simulink model "DAB_cc_2023a"  (R2023a)
settings: Solver=VariableStepAuto  StartTime=0.0  StopTime=0.3  RelTol=1e-3
undefined symbols (not defined in the file): Ion, Lithium
libraries: spsMosfetLib x8, spsVoltageMeasurementLib x6, spsSeriesRLCBranchLib x4, spsMeanLib x3, spsCurrentMeasurementLib x3, slpidlib x2, spsBatteryLib x1, spsDCVoltageSourceLib x1, spsLinearTransformerLib x1, spsRMSLib x1, eeGeneralControl x1, spspowerguiLib x1
settings Model: Creator=saivi  LastModifiedBy=saivi
settings RTWCC: GPUComputeCapability=5.0
settings ConfigComp: CovBoundaryAbsTol=1.0e-5

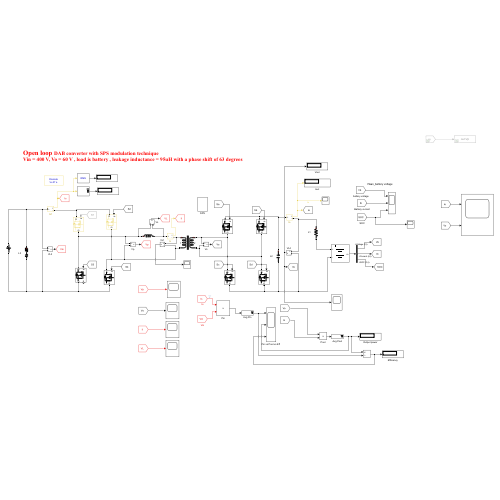
[thumbnail: Simulink's stored preview of the top-level diagram]
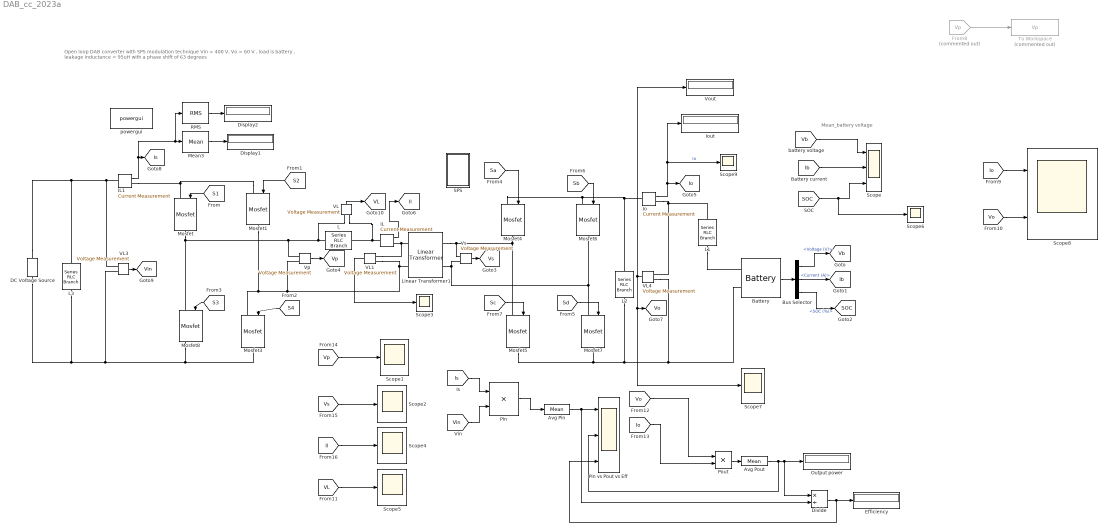
== system DAB_cc_2023a ==
  note: Open loop DAB converter with SPS modulation technique
      | Vin = 400 V, Vo = 60 V , load is battery , leakage inductance = 95uH with a phase shift of 63 degrees
  note: Mean_battery voltage
  Avg Pin : spsMeanLib/Mean  Freq=50000  Vinit=0  Ts=1e-7
  Avg Pout : spsMeanLib/Mean  Freq=50000  Vinit=0  Ts=1e-7
  Battery : spsBatteryLib/Battery  BatType=Lithium-Ion  NomV=48  NomQ=120  SOC=60  Batt_Tr=0.1  PresetModel=on  MaxQ=120  MinV=36  FullV=55.8714  Dis_rate=52.1739  R=0.004  Normal_OP=108.5217  expZone="[51.8585      5.89565]"
  Bus Selector : BusSelector  OutputSignals=Voltage (V),Current (A),SOC (%)
  DC Voltage Source : spsDCVoltageSourceLib/DC Voltage Source  Amplitude=400  Measurements=None
  Display1 : Display
  Display2 : Display
  Divide : Product  Inputs=*/
  Efficiency : Display
  From8 : From  Commented=on  GotoTag=Vp  TagVisibility=global
  IL : spsCurrentMeasurementLib/Current Measurement  PhasorSimulation=off  OutputType=Complex  PSBequivalent=0
  IL1 : spsCurrentMeasurementLib/Current Measurement  PhasorSimulation=off  OutputType=Complex  PSBequivalent=0
  Io : spsCurrentMeasurementLib/Current Measurement  PhasorSimulation=off  OutputType=Complex  PSBequivalent=0
  Iout : Display
  L : spsSeriesRLCBranchLib/Series RLC Branch  LConnTagsString=__new0  RConnTagsString=__new0  BranchType=L  Resistance=1  Inductance=90e-6  SetiL0=off  InitialCurrent=0  Capacitance=1e-6  Setx0=off  InitialVoltage=0  Measurements=None
  L1 : spsSeriesRLCBranchLib/Series RLC Branch  LConnTagsString=__new0  RConnTagsString=__new0  BranchType=R  Resistance=0.01  Inductance=19.108e-6*2  SetiL0=off  InitialCurrent=0  Capacitance=1000e-6  Setx0=off  InitialVoltage=0  Measurements=None
  L2 : spsSeriesRLCBranchLib/Series RLC Branch  LConnTagsString=__new0  RConnTagsString=__new0  BranchType=C  Resistance=0.8  Inductance=19.108e-6*2  SetiL0=off  InitialCurrent=0  Capacitance=1200e-6  Setx0=off  InitialVoltage=0  Measurements=None
  L3 : spsSeriesRLCBranchLib/Series RLC Branch  LConnTagsString=__new0  RConnTagsString=__new0  BranchType=RC  Resistance=0.8  Inductance=19.108e-6*2  SetiL0=off  InitialCurrent=0  Capacitance=1200e-6  Setx0=off  InitialVoltage=0  Measurements=None
  Linear Transformer1 : spsLinearTransformerLib/Linear Transformer  UNITS=SI  NominalPower=[1500 50000 ]  winding1=[400 0 0]  winding2=[60 0 0]  ThreeWindings=off  winding3=[3.15e+05 0.7938 0.084225]  RmLm=[5000 5866]  Measurements=None  DataType=on
  Mean3 : spsMeanLib/Mean  Freq=15000  Vinit=0  Ts=1e-6
  Mosfet{,1,3..7} (7 alike) : spsMosfetLib/Mosfet  Ron=0.01  Lon=0  Rd=0.01  Vfd=0  IC=0  Rs=1e5  Cs=inf  Measurements=off
  Mosfet8 : spsMosfetLib/Mosfet  Ron=0.01  Lon=0  Rd=0.01  Vfd=0  IC=0  Rs=1e5  Cs=inf  Measurements=on
  Output power : Display
  Pin : Product
  "Pin vs Pout vs Eff " : Scope  NumInputPorts=3
  Pout : Product
  RMS : spsRMSLib/RMS  TrueRMS=on  Freq=60  RMSInit=120  Ts=0
  SPS : Subsystem
  Scope : Scope  NumInputPorts=3
  Scope{1..7,9} (8 alike) : Scope
  Scope8 : Scope  NumInputPorts=2
  To Workspace : ToWorkspace  Commented=on  VariableName=Vp  SaveFormat=Structure With Time  SampleTime=-1
  VL{,1,3..4} (4 alike) : spsVoltageMeasurementLib/Voltage Measurement  PhasorSimulation=off  OutputType=Complex  PSBequivalent=0
  Vout : Display
  Vp : spsVoltageMeasurementLib/Voltage Measurement  PhasorSimulation=off  OutputType=Complex  PSBequivalent=0
  Vs : spsVoltageMeasurementLib/Voltage Measurement  PhasorSimulation=off  OutputType=Complex  PSBequivalent=0
  powergui : spspowerguiLib/powergui  Priority=1  SimulationMode=Discrete  SampleTime=1e-7  frequency=60  Iterations=50  frequencyindice=0  Pbase=100e6  ErrMax=1e-4  UnitsV=kV  UnitsW=MW  buscounter=0  FunctionMessages=off  echomessages=off  EnableUseOfTLC=off  CurrentSourceSwitches=off  DisableSnubberDevices=off  DisableRonSwitches=off  DisableVfSwitches=off  DisplayEquations=off  AutomaticDiscreteSolvers=off  SolverType=Tustin/Backward Euler (TBE)  Interpol=off  ExternalGateDelay=off  methode=off  Ts=100  x0status=blocks  SPID=on  SwTol=0  HookPort=off  NonlinearTolerance=1e-6  nMaxIteration=1000  ContinueOnMaxIteration=off  RestoreLinks=warning  ResistiveCurrentMeasurement=off  Frange=[0:2:500]  Ylog=off  Xlog=on  ShowGrid=off  save=off  variable=ZData  structure=0  ZoomFFT=off  StartTime=0.0  cycles=1  DisplayStyle=1  fundamental=60  FreqAxis=off  MaxFrequency=1000  frequencyindicesteady=1  RmsSteady=1  display=off
  tag scope: Ib=global, Il=global, Io=global, Is=global, SOC=global, VL=global, Vb=global, Vin=global, Vo=global, Vp=global, Vs=global
  wires:
  [Vs] -> Scope2/1
  [VL] -> Scope5/1
  [Vp] -> Scope1/1
  [Vin] -> Pin/2
  [Sb] -> Mosfet6/1
  Vs/1 -> [Vs]
  Battery/1 -> Bus Selector/1
  VL4/1 -> Scope7/1, [Vo], Vout/1
  [Sd] -> Mosfet7/1
  VL/1 -> [VL]
  RMS/1 -> Display2/1
  [S4] -> Mosfet3/1
  VL1/1 -> Scope3/1
  [Sc] -> Mosfet5/1
  [Is] -> Pin/1
  [Il] -> Scope4/1
  Mean3/1 -> Display1/1
  Bus Selector/3 -> [SOC]  "<SOC (%)>"
  IL1/1 -> RMS/1, Mean3/1, [Is]
  [Sa] -> Mosfet4/1
  Avg Pin/1 -> Divide/2, "Pin vs Pout vs Eff "/1
  [S2] -> Mosfet1/1
  From8/1 -> To Workspace/1
  [S3] -> Mosfet8/1
  Bus Selector/2 -> [Ib]  "<Current (A)>"
  [S1] -> Mosfet/1
  [Ib] -> Scope/2
  [Vo] -> Pout/1
  Pin/1 -> Avg Pin/1
  [Vb] -> Scope/1
  Avg Pout/1 -> "Pin vs Pout vs Eff "/2, Divide/1, Output power/1
  [SOC] -> Scope6/1, Scope/3
  Io/1 -> Iout/1, Scope9/1, [Io]  "Io"
  Vp/1 -> [Vp]
  Bus Selector/1 -> [Vb]  "<Voltage (V)>"
  IL/1 -> [Il]
  Divide/1 -> "Pin vs Pout vs Eff "/3, Efficiency/1
  VL3/1 -> [Vin]
  Pout/1 -> Avg Pout/1
  [Io] -> Pout/2
  [Io] -> Scope8/1
  [Vo] -> Scope8/2
  connections:
  Io/LConn1 -- Mosfet4/LConn1 -- Mosfet6/LConn1 -- L2/LConn1
  L/LConn1 -- VL/LConn1 -- Mosfet/RConn1 -- Mosfet8/LConn1 -- Vp/LConn1
  Mosfet6/RConn1 -- Mosfet7/LConn1 -- Vs/LConn2 -- Linear Transformer1/RConn2
  Linear Transformer1/LConn2 -- Vp/LConn2 -- Mosfet3/LConn1 -- Mosfet1/RConn1 -- VL1/LConn2
  L3/RConn1 -- Mosfet3/RConn1 -- Mosfet8/RConn1 -- VL3/LConn2 -- DC Voltage Source/LConn1
  DC Voltage Source/RConn1 -- VL3/LConn1 -- IL1/LConn1 -- L3/LConn1
  Mosfet1/LConn1 -- Mosfet/LConn1 -- IL1/RConn1
  Mosfet5/RConn1 -- Mosfet7/RConn1 -- VL4/LConn2 -- Battery/LConn2 -- L2/RConn1
  IL/RConn1 -- VL1/LConn1 -- Linear Transformer1/LConn1
  L/RConn1 -- IL/LConn1 -- VL/LConn2
  Mosfet4/RConn1 -- Mosfet5/LConn1 -- Linear Transformer1/RConn1 -- Vs/LConn1
  Io/RConn1 -- L1/LConn1 -- VL4/LConn1
  L1/RConn1 -- Battery/LConn1

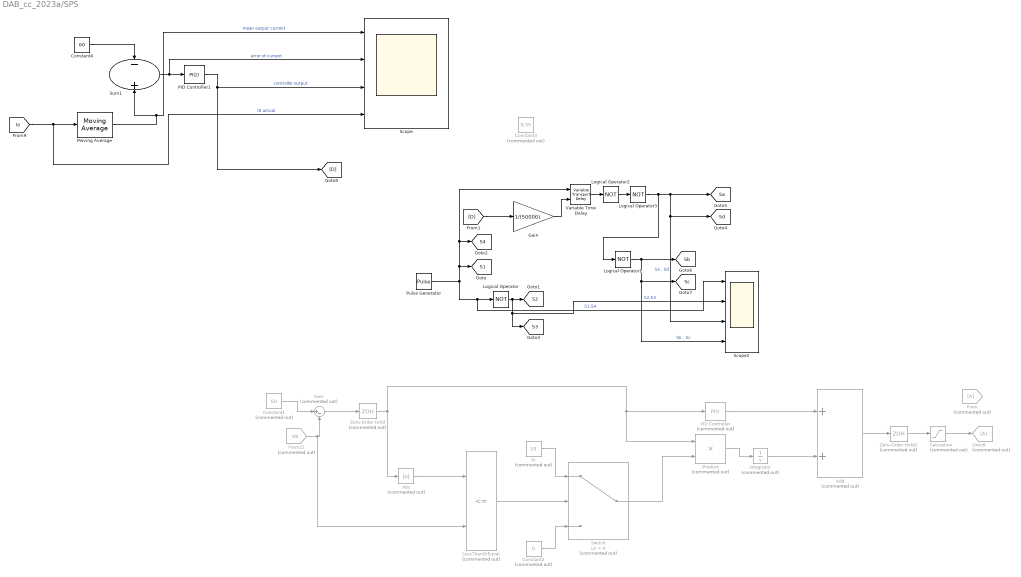
== system DAB_cc_2023a/SPS ==
  Abs : Abs  Commented=on  SaturateOnIntegerOverflow=off
  Add : Sum  Commented=on
  Constant1 : Constant  Commented=on  Value=60
  Constant2 : Constant  Commented=on  Value=0
  Constant3 : Constant  Commented=on  Value=0.35
  Constant4 : Constant  Value=60
  From : From  Commented=on
  From22 : From  Commented=on  GotoTag=Vb  TagVisibility=global
  Gain : Gain  Gain=1/(50000)
  Goto8 : Goto  Commented=on
  Integrator : Integrator  Commented=on
  Ki : Constant  Commented=on  Value=10
  LessThanOrEqual : RelationalOperator  Commented=on  Operator=<=  OutDataTypeStr=boolean  RndMeth=Simplest  InputSameDT=off
  Logical Operator{,1..3} (4 alike) : Logic  Operator=NOT  AllPortsSameDT=off  OutDataTypeStr=boolean
  Moving Average : eeGeneralControl/Moving Average  VariantControl=Variant1  LabelModeActiveChoice=Discrete  f=50000  x0=0  BufferSize=8192  Ts=1e-7
      settings: LibrarySourceBlock=ee_sl_lib/General Control/Moving Average
  PID Controller : slpidlib/PID Controller  Commented=on  Controller=P  Form=Parallel  TimeDomain=Continuous-time  UseExternalTs=off  SampleTime=-1  IntegratorMethod=Forward Euler  FilterMethod=Forward Euler  ControllerParametersSource=internal  P=0.05  I=1  UseKiTs=off  D=0  N=100  UseFilter=on  TunerSelectOption=Transfer Function Based (PID Tuner App)  InitialConditionSource=internal  InitialConditionForIntegrator=0  InitialConditionForFilter=0  DifferentiatorICPrevScaledInput=0  ExternalReset=none  TrackingMode=off  Kt=1  LimitOutput=off  SatLimitsSource=internal  UpperSaturationLimit=inf  LowerSaturationLimit=-inf  LinearizeAsGain=on  AntiWindupMode=none  Kb=1  LimitIntegrator=off  UpperIntegratorSaturationLimit=inf  LowerIntegratorSaturationLimit=-inf  POutMin=[]  POutMax=[]  IOutMin=[]  IOutMax=[]  DOutMin=[]  DOutMax=[]  NOutMin=[]  NOutMax=[]  SumOutMin=[]  SumOutMax=[]  SaturationOutMin=[]  SaturationOutMax=[]  PParamMin=[]  PParamMax=[]  IParamMin=[]  IParamMax=[]  DParamMin=[]  DParamMax=[]  NParamMin=[]  NParamMax=[]  KbParamMin=[]  KbParamMax=[]  KtParamMin=[]  KtParamMax=[]  KbOutMin=[]  KbOutMax=[]  KtOutMin=[]  KtOutMax=[]  IntegratorOutMin=[]  IntegratorOutMax=[]  FilterOutMin=[]  FilterOutMax=[]  SumI1OutMin=[]  SumI1OutMax=[]  SumI2OutMin=[]  SumI2OutMax=[]  SumI3OutMin=[]  SumI3OutMax=[]  SumI4OutMin=[]  SumI4OutMax=[]  SumDOutMin=[]  SumDOutMax=[]  DifferentiatorOutMin=[]  DifferentiatorOutMax=[]  FilterDiffOutCoefMin=[]  FilterDiffOutCoefMax=[]  ReciprocalOutMin=[]  ReciprocalOutMax=[]  SumDenOutMin=[]  SumDenOutMax=[]  SumNumOutMin=[]  SumNumOutMax=[]  DivideOutMin=[]  DivideOutMax=[]  UdiffTsProdOutMin=[]  UdiffTsProdOutMax=[]  NTsProdOutMin=[]  NTsProdOutMax=[]  UintegralTsProdOutMin=[]  UintegralTsProdOutMax=[]  UngainTsProdOutMin=[]  UngainTsProdOutMax=[]  ClampingZeroOutDataTypeStr=Inherit: Inherit via back propagation  ClampingZeroOutMin=[]  ClampingZeroOutMax=[]  FilterDenConstantOutDataTypeStr=Inherit: Inherit via back propagation  FilterDenConstantOutMin=[]  FilterDenConstantOutMax=[]  PCopyOutDataTypeStr=Inherit: Inherit via back propagation  PCopyOutMin=[]  PCopyOutMax=[]  NCopyOutDataTypeStr=Inherit: Inherit via back propagation  NCopyOutMin=[]  NCopyOutMax=[]  IntegratorContinuousStateAttributes=''  IntegratorStateMustResolveToSignalObject=off  IntegratorRTWStateStorageClass=Auto  FilterContinuousStateAttributes=''  FilterStateMustResolveToSignalObject=off  FilterRTWStateStorageClass=Auto  ParallelPVariant=InternalParameters  IdealPVariant=Disabled  IVariant=Disabled  DVariant=Disabled  IntegratorVariant=Disabled  SatVariant=Disabled  AWVariant=Disabled  PCopyVariant=Disabled  TRVariant=Disabled  FdbkBlocksVariant=Forward  IdealPFdbkVariant=Disabled  SatFdbkVariant=Disabled  DerivativeFilterVariant=Disabled  NVariant=Disabled  NCopyVariant=Disabled_SignalSpec  FilterICVariant=Disabled  IntegratorICVariant=Disabled  ExternalResetVariant=Disabled  TRSumVariant=Passthrough  SumFdbkVariant=Disabled  SumVariant=Passthrough_P  TsampFilterVariant=InternalTs  TsampNgainVariant=Passthrough  TsampIntegralVariant=Disabled_SignalSpec  ExternalSaturationOutDataTypeStr=Inherit: Same as second input
  PID Controller1 : slpidlib/PID Controller  Controller=PI  Form=Parallel  TimeDomain=Discrete-time  UseExternalTs=off  SampleTime=20e-6  IntegratorMethod=Forward Euler  FilterMethod=Forward Euler  ControllerParametersSource=internal  P=0.1252  I=2000  UseKiTs=off  D=0  N=100  UseFilter=on  TunerSelectOption=Transfer Function Based (PID Tuner App)  InitialConditionSource=internal  InitialConditionForIntegrator=0.35  InitialConditionForFilter=0  DifferentiatorICPrevScaledInput=0  ExternalReset=none  TrackingMode=off  Kt=1  LimitOutput=on  SatLimitsSource=internal  UpperSaturationLimit=0.5  LowerSaturationLimit=0.111  LinearizeAsGain=on  AntiWindupMode=back-calculation  Kb=1  LimitIntegrator=off  UpperIntegratorSaturationLimit=inf  LowerIntegratorSaturationLimit=-inf  POutMin=[]  POutMax=[]  IOutMin=[]  IOutMax=[]  DOutMin=[]  DOutMax=[]  NOutMin=[]  NOutMax=[]  SumOutMin=[]  SumOutMax=[]  SaturationOutMin=[]  SaturationOutMax=[]  PParamMin=[]  PParamMax=[]  IParamMin=[]  IParamMax=[]  DParamMin=[]  DParamMax=[]  NParamMin=[]  NParamMax=[]  KbParamMin=[]  KbParamMax=[]  KtParamMin=[]  KtParamMax=[]  KbOutMin=[]  KbOutMax=[]  KtOutMin=[]  KtOutMax=[]  IntegratorOutMin=[]  IntegratorOutMax=[]  FilterOutMin=[]  FilterOutMax=[]  SumI1OutMin=[]  SumI1OutMax=[]  SumI2OutMin=[]  SumI2OutMax=[]  SumI3OutMin=[]  SumI3OutMax=[]  SumI4OutMin=[]  SumI4OutMax=[]  SumDOutMin=[]  SumDOutMax=[]  DifferentiatorOutMin=[]  DifferentiatorOutMax=[]  FilterDiffOutCoefMin=[]  FilterDiffOutCoefMax=[]  ReciprocalOutMin=[]  ReciprocalOutMax=[]  SumDenOutMin=[]  SumDenOutMax=[]  SumNumOutMin=[]  SumNumOutMax=[]  DivideOutMin=[]  DivideOutMax=[]  UdiffTsProdOutMin=[]  UdiffTsProdOutMax=[]  NTsProdOutMin=[]  NTsProdOutMax=[]  UintegralTsProdOutMin=[]  UintegralTsProdOutMax=[]  UngainTsProdOutMin=[]  UngainTsProdOutMax=[]  ClampingZeroOutDataTypeStr=Inherit: Inherit via back propagation  ClampingZeroOutMin=[]  ClampingZeroOutMax=[]  FilterDenConstantOutDataTypeStr=Inherit: Inherit via back propagation  FilterDenConstantOutMin=[]  FilterDenConstantOutMax=[]  PCopyOutDataTypeStr=Inherit: Inherit via back propagation  PCopyOutMin=[]  PCopyOutMax=[]  NCopyOutDataTypeStr=Inherit: Inherit via back propagation  NCopyOutMin=[]  NCopyOutMax=[]  IntegratorContinuousStateAttributes=''  IntegratorStateMustResolveToSignalObject=off  IntegratorRTWStateStorageClass=Auto  FilterContinuousStateAttributes=''  FilterStateMustResolveToSignalObject=off  FilterRTWStateStorageClass=Auto  ParallelPVariant=InternalParameters  IdealPVariant=Disabled  IVariant=InternalParameters  DVariant=Disabled  IntegratorVariant=Discrete  SatVariant=Enabled  AWVariant=BackCalculation  PCopyVariant=Disabled  TRVariant=Disabled  FdbkBlocksVariant=Forward  IdealPFdbkVariant=Disabled  SatFdbkVariant=Disabled  DerivativeFilterVariant=Disabled  NVariant=Disabled  NCopyVariant=Disabled_SignalSpec  FilterICVariant=Disabled  IntegratorICVariant=InternalICs  ExternalResetVariant=Disabled  TRSumVariant=Passthrough  SumFdbkVariant=Disabled  SumVariant=Sum_PI  TsampFilterVariant=InternalTs  TsampNgainVariant=Passthrough  TsampIntegralVariant=Disabled_SignalSpec  ExternalSaturationOutDataTypeStr=Inherit: Same as second input
  Product : Product  Commented=on
  Pulse Generator : DiscretePulseGenerator  PulseType=Time based  Period=1/50000  PulseWidth=50
  Saturation : Saturate  Commented=on
  Scope : Scope  NumInputPorts=4
  Scope2 : Scope  NumInputPorts=4
  Sum : Sum  Commented=on  Inputs=|+-
  Sum1 : Sum  Inputs=-+
  Switch : Switch  Commented=on  Criteria=u2 > Threshold  SaturateOnIntegerOverflow=off  InputSameDT=off
  Variable Time Delay : VariableTransportDelay  MaximumDelay=10
  Zero-Order Hold : ZeroOrderHold  Commented=on  SampleTime=-1
  Zero-Order Hold1 : ZeroOrderHold  Commented=on  SampleTime=-1
  tag scope: S1=global, S2=global, S3=global, S4=global, Sa=global, Sb=global, Sc=global, Sd=global
  wires:
  Variable Time Delay/1 -> Logical Operator2/1
  Logical Operator1/1 -> Scope2/4, [Sc], [Sb]  "Sb , Sc"
  Pulse Generator/1 -> Variable Time Delay/1, [S4], [S1], Scope2/1, Logical Operator/1  "S1,S4"
  Logical Operator/1 -> [S3], Scope2/2, [S2]  "S2,S3"
  Gain/1 -> Variable Time Delay/2
  Logical Operator2/1 -> Logical Operator3/1
  Logical Operator3/1 -> Logical Operator1/1, [Sa], Scope2/3, [Sd]  "Sa , Sd"
  Constant1/1 -> Sum/1
  From22/1 -> LessThanOrEqual/2, Sum/2
  Sum/1 -> Zero-Order Hold/1
  Zero-Order Hold/1 -> Abs/1, Product/1, PID Controller/1
  PID Controller/1 -> Add/1
  Abs/1 -> LessThanOrEqual/1
  LessThanOrEqual/1 -> Switch/2
  Ki/1 -> Switch/1
  Constant2/1 -> Switch/3
  Switch/1 -> Product/2
  Product/1 -> Integrator/1
  Integrator/1 -> Add/2
  Add/1 -> Zero-Order Hold1/1
  Zero-Order Hold1/1 -> Saturation/1
  Saturation/1 -> Goto8/1
  Constant4/1 -> Sum1/1
  Sum1/1 -> Scope/2, PID Controller1/1  "error of current"
  PID Controller1/1 -> [D], Scope/3  "controller output"
  [Io] -> Scope/4, Moving Average/1  "I0 actual"
  Moving Average/1 -> Sum1/2, Scope/1  "mean output current"
  [D] -> Gain/1
